simulink model "final"  (R2024a)
settings: Solver=ode5  StartTime=0.0  StopTime=20  RelTol=1e-3
libraries: instrumentlib x1
settings Model: Creator=divya  LastModifiedBy=divya
settings HardwareCC: ProdBitPerLong=64  ProdHWDeviceType=Intel->x86-64 (Linux 64)
settings RTWCC: Description=Simulink Desktop Real-Time  SystemTargetFile=sldrt.tlc  TemplateMakefile=sldrt.tmf  RTWCompilerOptimization=on
settings CodeAppCC: MaxIdLength=95
settings SimulinkDesktopRealTimeCC: TargetLibSuffix=_sldrt.a  TargetPreCompLibLocation=D:\matlab\toolbox\sldrt\lib\win64

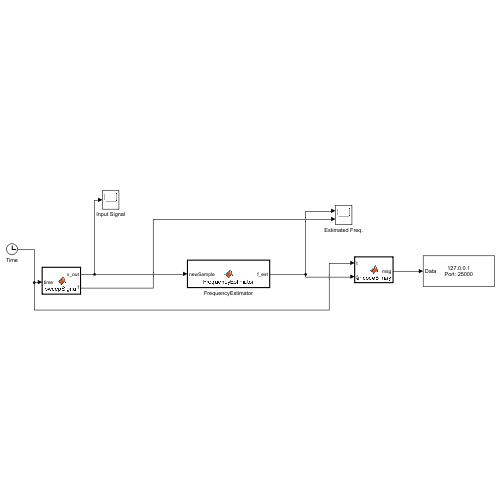
[thumbnail: Simulink's stored preview of the top-level diagram]
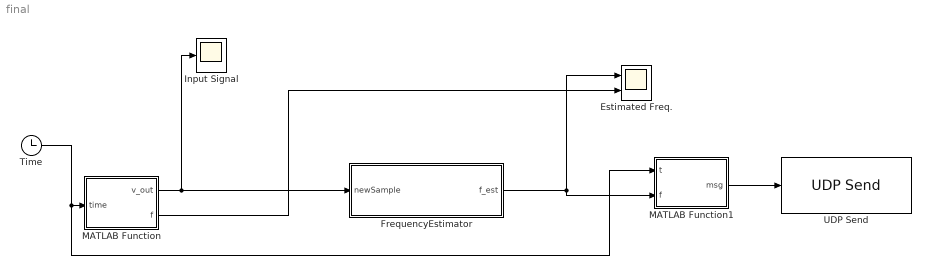
== system final ==
  Estimated Freq. : Scope  NumInputPorts=2
  FrequencyEstimator : MATLAB Function  TreatAsAtomicUnit=on  SystemSampleTime=0.000625
  Input Signal : Scope
  MATLAB Function : MATLAB Function  TreatAsAtomicUnit=on  SystemSampleTime=0.000005
  MATLAB Function1 : MATLAB Function  TreatAsAtomicUnit=on  SystemSampleTime=0.1
  Time : Clock
  UDP Send : instrumentlib/UDP Send  Host=127.0.0.1  Port=25000  LocalAddress=0.0.0.0  LocalPort=-1  EnablePortSharing=off  OutputDatagramPacketSize=512  ByteOrder=big-endian  EnableBlockingMode=on  SimulateUsing=Interpreted execution
  wires:
  Time/1 -> MATLAB Function1/1(t), MATLAB Function/1(time)
  MATLAB Function/2(f) -> Estimated Freq./2
  MATLAB Function/1(v_out) -> Input Signal/1, FrequencyEstimator/1(newSample)
  FrequencyEstimator/1(f_est) -> Estimated Freq./1, MATLAB Function1/2(f)
  MATLAB Function1/1(msg) -> UDP Send/1

== matlab function final/MATLAB Function ==
  data: time input; v_out output; f output
function [v_out,f] = sweepSignal(time)
%#codegen
% v(t) = sin(ω(t)*t)
%      + 0.0856*sin(5*ω(t)*t)
%      + …

% ω(t) sweeps 51→49 Hz over 0≤t<0.27 s,
% holds at 49 Hz for 0.27≤t<0.54 s,
% sweeps back 49→51 Hz over 0.54≤t<0.81 s,
% then holds at 51 Hz for t≥0.81 s.

if time < 10
    f = 50;       % 51→49 over 0.27 s
elseif time < 20
    f = 51;                       % hold
else
    f = 50;
end

omega0 = 2*pi * f;

v_out = sin(omega0 * time) + ...
        0.0856 * sin(5 * omega0 * time) + ...
        0.0428 * sin(7 * omega0 * time) + ...
        0*0.0306 * sin(11 * omega0 * time) + ...
        0*0.0183 * sin(13 * omega0 * time);
end

== matlab function final/MATLAB Function1 ==
  data: t input; msg output; f input
function msg = encodeBinary(t, f)
%#codegen

  % Create an array of two doubles and typecast to bytes
  data = [t, f];
  msg = typecast(data, 'uint8');
end

== matlab function final/FrequencyEstimator ==
  data: newSample input; f_est output
function f_est = FrequencyEstimator(newSample)
    persistent buffer sampleCount Ts N_window f_prev allowed_harmonics
    if isempty(sampleCount)
        Ts = 1/1600;
        N_window = 16;
        buffer = zeros(N_window,1);
        sampleCount = 0;
        f_prev = 50;
        allowed_harmonics = [1,5,7,11,13];
    end

    if sampleCount < N_window
        sampleCount = sampleCount + 1;
        buffer(sampleCount) = newSample;
        f_est = f_prev;
        return;
    else
        buffer(1:end-1) = buffer(2:end);
        buffer(end)     = newSample;
    end

    t_window = (0:N_window-1)' * Ts;
    x_vals   = 48.5:0.1:51.5;           % frequency grid
    n        = length(x_vals);

    % build Fibonacci sequence up to >= n
    fib = [1, 1];
    while fib(end) < n
        fib(end+1) = fib(end) + fib(end-1);
    end
    k     = numel(fib) - 1;
    a_idx = 1;
    b_idx = n;

    % discrete Fibonacci search loop
    while k > 0
        mid = a_idx + fib(k) - 1;
        if mid >= b_idx
            mid = b_idx - 1;
        end

        % compute the two errors
        err1 = compute_err(buffer, t_window, allowed_harmonics, x_vals(mid));
        err2 = compute_err(buffer, t_window, allowed_harmonics, x_vals(mid+1));

        if err1 < err2
            b_idx = mid;      % minimum is in [a_idx, mid]
            k     = k - 1;
        else
            a_idx = mid + 1;  % minimum is in [mid+1, b_idx]
            k     = k - 2;
        end
    end

    f_prev = x_vals(a_idx);
    f_est  = f_prev;
end

function err = compute_err(buffer, t_window, allowed_harmonics, f)
    % build the regression matrix M
    M = zeros(numel(buffer), numel(allowed_harmonics)*2);
    col = 1;
    for hh = allowed_harmonics
        M(:,col) = cos(2*pi*f*hh*t_window);
        col = col + 1;
    end
    for hh = allowed_harmonics
        M(:,col) = sin(2*pi*f*hh*t_window);
        col = col + 1;
    end

    % least-squares fit and error
    coeff      = (M'*M)\(M'*buffer);
    buffer_est = M * coeff;
    err        = sum((buffer - buffer_est).^2);
end
